simulink model "cav_adas_AutomatedDrivingToolbox"  (R2022a)
settings: Solver=VariableStepAuto  StartTime=0.0  StopTime=500  MaxStep=1e-1  RelTol=1e-3
values from neighbouring files (symbols this model uses):
  Af = 2.33    [data_cav.m]
  Cd = 0.28    [data_cav.m]
  elev_date_1 = date_elev(:,1)    [data_cav.m]
  elev_date_2 = date_elev(:,2)    [data_cav.m]
  eta = 0.93    [data_cav.m]
  fr = 0.015    [data_cav.m]
  g = 9.81    [data_cav.m]
  m = 1521    [data_cav.m]
  R = 0.5    [data_cav.m]
  rho = 1.2    [data_cav.m]
  slope_date_1 = date_slope(:,1)    [data_cav.m]
  slope_date_2_degree = zeros(length(slope_date_2_grad),1)    [data_cav.m]
libraries: sim3dautolib x2, drivingscenarioandsensors x2, mpclib x1, sim3dlib x1
settings Model: Creator=user  LastModifiedBy=user

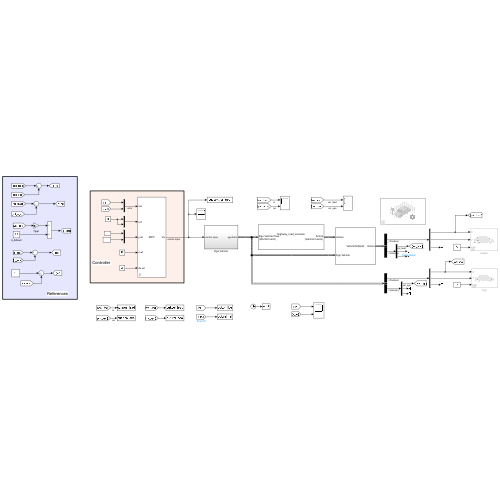
[thumbnail: Simulink's stored preview of the top-level diagram]
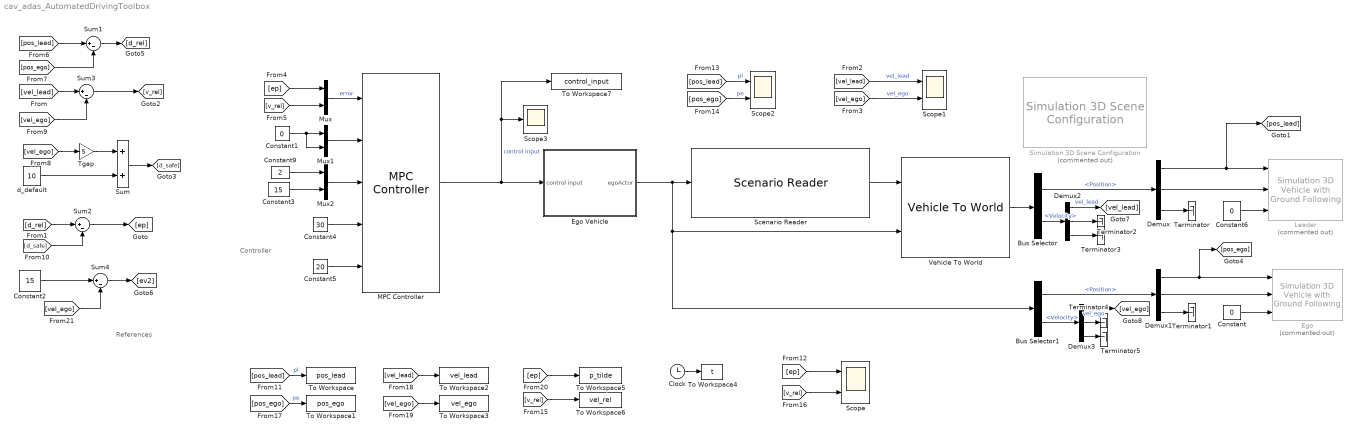
== system cav_adas_AutomatedDrivingToolbox ==
  note: Controller
  note: References
  Bus Selector : BusSelector  OutputSignals=Actors.Position,Actors.Velocity
  Bus Selector1 : BusSelector  OutputSignals=Position,Velocity
  Clock : Clock
  Constant : Constant  Value=0
  Constant1 : Constant  Value=0
  Constant2 : Constant  Value=15
  Constant3 : Constant  Value=15
  Constant4 : Constant  Value=30
  Constant5 : Constant  Value=20
  Constant6 : Constant  Value=0
  Constant9 : Constant  Value=2
  Demux{,1..3} (4 alike) : Demux  Outputs=3
  Ego : sim3dautolib/Simulation 3D Vehicle with Ground Following  Priority=-1  Commented=on  PassVehMesh=Sport utility vehicle  MeshPath=/MathWorksSimulation/Vehicles/Muscle/Meshes/SK_MuscleCar.SK_MuscleCar  TrackWidth=1.9  WheelBase=3  WheelRadius=0.35  VehColor=Blue  InitialPos=[0, 0, 0]  InitialRot=[0, 0, 0]  ActorName=EgoVehicle  SampleTime=-1  ActorType=SimulinkVehicle  ID=C  aMode=3  ActorTag=EgoVehicle  CoordinateScheme=ISO  VehLightsControl=off  HeadlightColor=[ 1, 1, 1 ]  HighBeamIntensity=100000  LowBeamIntensity=60000  HighBeamConeAngle=70  LowBeamConeAngle=70  LeftHeadlightOrientation=[ 0, 0 ]  RightHeadlightOrientation=[ 0, 0 ]  BrakelightIntensity=500  ReverselightIntensity=500  SignallightIntensity=500  SignallightPeriod=1  SignalPulseWidth=50  TransformOutportEnabled=off
      settings: SourceProductBaseCode=VE,AE,DR,UV,VE
  Ego Vehicle : Subsystem
  Leader : sim3dautolib/Simulation 3D Vehicle with Ground Following  Priority=-1  Commented=on  PassVehMesh=Muscle car  MeshPath=/MathWorksSimulation/Vehicles/Muscle/Meshes/SK_MuscleCar.SK_MuscleCar  TrackWidth=1.9  WheelBase=3  WheelRadius=0.35  VehColor=Red  InitialPos=[0, 0, 0]  InitialRot=[0, 0, 0]  ActorName=LeaderVehicle  SampleTime=-1  ActorType=SimulinkVehicle  ID=C  aMode=3  ActorTag=LeaderVehicle  CoordinateScheme=ISO  VehLightsControl=off  HeadlightColor=[ 1, 1, 1 ]  HighBeamIntensity=100000  LowBeamIntensity=60000  HighBeamConeAngle=70  LowBeamConeAngle=70  LeftHeadlightOrientation=[ 0, 0 ]  RightHeadlightOrientation=[ 0, 0 ]  BrakelightIntensity=500  ReverselightIntensity=500  SignallightIntensity=500  SignallightPeriod=1  SignalPulseWidth=50  TransformOutportEnabled=off
      settings: SourceProductBaseCode=VE,AE,DR,UV,VE
  MPC Controller : mpclib/MPC Controller  SCDEnableBlockLinearizationSpecification=on  mpcobj=mpc1  is_multiple=0  enable_value=0  return_u0=off  updateMPCinCallerWorkspace=on  md_inport=off  mv_inport=off  uref_inport=off  return_cost=off  return_mvseq=off  return_qpstatus=off  return_xseq=off  return_state=off  return_ovseq=off  state_inport=off  umin_inport=off  umax_inport=off  ymin_inport=off  ymax_inport=off  cc_inport=off  ywt_inport=on  uwt_inport=on  duwt_inport=on  rhoeps_inport=off  pm_inport=off  MaximumP=10  HorizonChoice=FixedHorizon  n_ts=0.1  n_p=50  n_mv=1  n_md=0  n_ud=0  n_mo=2  n_uo=0  BlockDataType=double  SampleTimeInherited=off  switch_inport=off
  Mux : Mux  Inputs=2
  Mux1 : Mux  Inputs=2
  Mux2 : Mux  Inputs=2
  Scenario Reader : drivingscenarioandsensors/Scenario Reader  ScenarioSource=From file  ScenarioFileName=D:\Università\MAGISTRALE\CSAGV\Challenge 2022\MATLAB & Simulink Files\Highway_road_scenario.mat  ScenarioVariableName=scenario  OutputCoordinateSystem=Vehicle coordinates  EgoVehicleSource=Input port  EgoVehicleActorID=1  OrientVehiclesOnRoad=off  OutputEgoVehiclePose=off  OutputEgoVehicleState=off  SampleTime=0.1  LaneBoundaryOutput=None  LaneBoundaryDistance=0:0.5:9.5  LaneBoundaryLocation=Center of lane markings  BusNameSource=Auto  BusName=BusActors  BusNumActorsSource=Scenario  BusNumActors=100  BusName2Source=Auto  BusName2=BusLaneBoundaries  BusNumLaneBoundariesSource=Scenario  BusNumLaneBoundaries=10  BusName3Source=Auto  BusName3=BusEgoActor  BusName4Source=Auto  BusName4=BusEgoState  ShowCoordinateLabels=on  SimulateUsing=Interpreted execution
  Scope : Scope  NumInputPorts=2
  Scope1 : Scope  NumInputPorts=2
  Scope2 : Scope  NumInputPorts=2
  Scope3 : Scope
  Simulation 3D Scene Configuration : sim3dlib/Simulation 3D Scene Configuration  Priority=0  Commented=on  ProjectFormat=Default Scenes  SceneDesc=Straight road  ProjectName=C:\Program Files\MATLAB\R2022a\toolbox\shared\sim3d_projects\automotive_project\UE4\WindowsNoEditor\VehicleSimulation.exe  ScenePath=/Game/Maps/HwStrght  vehTagList={'EgoVehicle';'LeaderVehicle';'Scene Origin'}  vehTag=EgoVehicle  OpVisEn=off  Ts=1/60  EnableWindow=on  EnableRemoteAccess=off  EnableWeather=off  SunAltitude=40.0  SunAzimuth=90  clouds=10  wind=1  fog=0  rain=0  sensorTag=MainCamera1  sensorId=1  sensorName=MainCamera1  mountLoc=Origin  offsetFlag=off  tmountOffset=[0, 0, 0]  rmountOffset=[0, 0, 0]  HorizontalResolution=1280  VerticalResolution=720  HorizontalFOV=60  mountPoint=[0 0 0]  mountOrientation=[0 0 0]  aMode=3  ID=1
      settings: SourceProductBaseCode=VE,AE,DR,UV,VE
  Sum : Sum
  Sum{1..4} (4 alike) : Sum  Inputs=|+-
  Terminator{,1..5} (6 alike) : Terminator
  Tgap : Gain  Gain=5
  To Workspace : ToWorkspace  VariableName=pos_lead  SampleTime=-1
      settings: Save2DSignal=2-D array (concatenate along first dimension)
  To Workspace1 : ToWorkspace  VariableName=pos_ego  SampleTime=-1
      settings: Save2DSignal=2-D array (concatenate along first dimension)
  To Workspace2 : ToWorkspace  VariableName=vel_lead  SampleTime=-1
      settings: Save2DSignal=2-D array (concatenate along first dimension)
  To Workspace3 : ToWorkspace  VariableName=vel_ego  SampleTime=-1
      settings: Save2DSignal=2-D array (concatenate along first dimension)
  To Workspace4 : ToWorkspace  VariableName=t  SampleTime=-1
      settings: Save2DSignal=2-D array (concatenate along first dimension)
  To Workspace5 : ToWorkspace  VariableName=p_tilde  SampleTime=-1
      settings: Save2DSignal=2-D array (concatenate along first dimension)
  To Workspace6 : ToWorkspace  VariableName=vel_rel  SampleTime=-1
      settings: Save2DSignal=2-D array (concatenate along first dimension)
  To Workspace7 : ToWorkspace  VariableName=control_input  SampleTime=-1
      settings: Save2DSignal=2-D array (concatenate along first dimension)
  Vehicle To World : drivingscenarioandsensors/Vehicle To World  BusNameSource=Auto  BusName=BusVehicleToWorldActors  SimulateUsing=Interpreted execution
      settings: SourceProductBaseCode=DR
  d_default : Constant  Value=10
  wires:
  Mux1/1 -> MPC Controller/2
  [d_safe] -> Sum2/2
  [d_rel] -> Sum2/1
  Sum2/1 -> [ep]
  Sum/1 -> [d_safe]
  Mux2/1 -> MPC Controller/3
  [ep] -> Mux/1
  d_default/1 -> Sum/2
  Constant1/1 -> Mux1/2, Mux1/1
  Constant3/1 -> Mux2/2
  Constant5/1 -> MPC Controller/5
  [vel_ego] -> Sum3/2
  Tgap/1 -> Sum/1
  Sum3/1 -> [v_rel]
  Mux/1 -> MPC Controller/1  "error"
  [vel_ego] -> Tgap/1
  [pos_lead] -> Scope2/1  "pl"
  Constant4/1 -> MPC Controller/4
  [pos_ego] -> Sum1/2
  [vel_ego] -> Scope1/2  "vel_ego"
  [vel_lead] -> Scope1/1  "vel_lead"
  Sum1/1 -> [d_rel]
  [pos_ego] -> Scope2/2  "pe"
  Ego Vehicle/1(egoActor) -> Bus Selector1/1, Vehicle To World/2, Scenario Reader/1
  Scenario Reader/1 -> Vehicle To World/1
  Vehicle To World/1 -> Bus Selector/1
  Bus Selector/1 -> Demux/1  "<Position>"
  Bus Selector1/1 -> Demux1/1  "<Position>"
  Constant/1 -> Ego/3
  Constant6/1 -> Leader/3
  Demux/3 -> Terminator/1
  Demux/1 -> Leader/1, [pos_lead]
  Demux/2 -> Leader/2
  Demux1/3 -> Terminator1/1
  Demux1/1 -> Ego/1, [pos_ego]
  Demux1/2 -> Ego/2
  Bus Selector/2 -> Demux2/1  "<Velocity>"
  Bus Selector1/2 -> Demux3/1  "<Velocity>"
  Demux2/1 -> [vel_lead]  "vel_lead"
  Demux2/2 -> Terminator2/1
  Demux2/3 -> Terminator3/1
  Demux3/2 -> Terminator4/1
  Demux3/3 -> Terminator5/1
  Demux3/1 -> [vel_ego]  "vel_ego"
  MPC Controller/1 -> Scope3/1, To Workspace7/1, Ego Vehicle/1(control input)  "control input"
  [vel_lead] -> Sum3/1
  [pos_lead] -> Sum1/1
  [v_rel] -> Mux/2
  Constant9/1 -> Mux2/1
  [v_rel] -> To Workspace6/1
  [pos_ego] -> To Workspace1/1  "pe"
  [pos_lead] -> To Workspace/1  "pl"
  [vel_ego] -> To Workspace3/1
  [ep] -> To Workspace5/1
  [vel_lead] -> To Workspace2/1
  Clock/1 -> To Workspace4/1
  [v_rel] -> Scope/2
  [ep] -> Scope/1
  Sum4/1 -> [ev2]
  Constant2/1 -> Sum4/1
  [vel_ego] -> Sum4/2

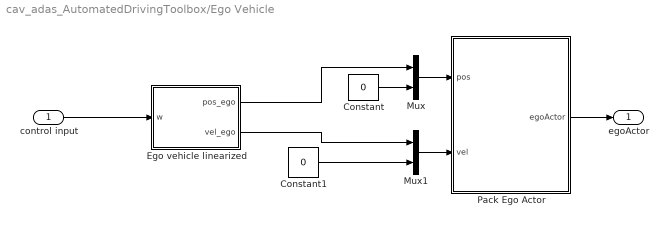
== system cav_adas_AutomatedDrivingToolbox/Ego Vehicle ==
  control input : Inport
  Constant : Constant  Value=0
  Constant1 : Constant  Value=0
  Ego vehicle linearized : Subsystem
  Mux : Mux  Inputs=2
  Mux1 : Mux  Inputs=2
  Pack Ego Actor : MATLAB Function  TreatAsAtomicUnit=on
  egoActor : Outport
  wires:
  control input/1 -> Ego vehicle linearized/1(w)
  Pack Ego Actor/1(egoActor) -> egoActor/1
  Mux/1 -> Pack Ego Actor/1(pos)
  Mux1/1 -> Pack Ego Actor/2(vel)
  Ego vehicle linearized/1(pos_ego) -> Mux/1
  Ego vehicle linearized/2(vel_ego) -> Mux1/1
  Constant1/1 -> Mux1/2
  Constant/1 -> Mux/2

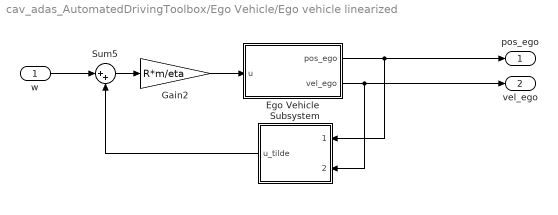
== system cav_adas_AutomatedDrivingToolbox/Ego Vehicle/Ego vehicle linearized ==
  w : Inport
  "Ego Vehicle " : Subsystem
  Gain2 : Gain  Gain=R*m/eta
  Subsystem : Subsystem
  Sum5 : Sum  Inputs=|++
  pos_ego : Outport
  vel_ego : Outport  Port=2
  wires:
  "Ego Vehicle "/2(vel_ego) -> vel_ego/1, Subsystem/2(vel_ego)
  "Ego Vehicle "/1(pos_ego) -> pos_ego/1, Subsystem/1(pos_ego)
  Sum5/1 -> Gain2/1
  w/1 -> Sum5/1
  Gain2/1 -> "Ego Vehicle "/1(u)
  Subsystem/1(u_tilde) -> Sum5/2

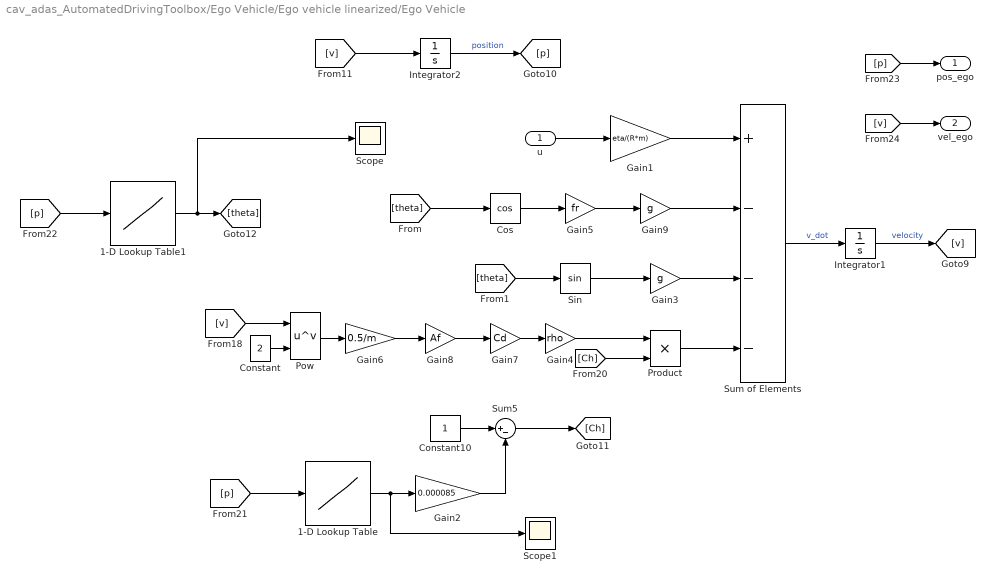
== system cav_adas_AutomatedDrivingToolbox/Ego Vehicle/Ego vehicle linearized/Ego Vehicle  ==
  u : Inport
  1-D Lookup Table : Lookup_n-D  NumberOfTableDimensions=1  BreakpointsForDimension1=elev_date_1  Table=elev_date_2  InternalRulePriority=Speed  RndMeth=Simplest
  1-D Lookup Table1 : Lookup_n-D  NumberOfTableDimensions=1  BreakpointsForDimension1=slope_date_1  Table=slope_date_2_degree  InternalRulePriority=Speed  RndMeth=Simplest
  Constant : Constant  Value=2
  Constant10 : Constant
  Cos : Trigonometry  Operator=cos
  Gain1 : Gain  Gain=eta/(R*m)
  Gain2 : Gain  Gain=0.000085
  Gain3 : Gain  Gain=g
  Gain4 : Gain  Gain=rho
  Gain5 : Gain  Gain=fr
  Gain6 : Gain  Gain=0.5/m
  Gain7 : Gain  Gain=Cd
  Gain8 : Gain  Gain=Af
  Gain9 : Gain  Gain=g
  Integrator1 : Integrator
  Integrator2 : Integrator
  Pow : Math  Operator=pow  RndMeth=Zero
  Product : Product
  Scope : Scope
  Scope1 : Scope
  Sin : Trigonometry
  Sum of Elements : Sum  Inputs=+---
  Sum5 : Sum  Inputs=|+-
  pos_ego : Outport
  vel_ego : Outport  Port=2
  wires:
  [p] -> 1-D Lookup Table/1
  1-D Lookup Table1/1 -> Scope/1, [theta]
  Gain5/1 -> Gain9/1
  Gain6/1 -> Gain8/1
  [Ch] -> Product/2
  Sin/1 -> Gain3/1
  Gain4/1 -> Product/1
  Sum5/1 -> [Ch]
  Gain1/1 -> Sum of Elements/1
  Integrator2/1 -> [p]  "position"
  Constant10/1 -> Sum5/1
  Gain9/1 -> Sum of Elements/2
  Integrator1/1 -> [v]  "velocity"
  Pow/1 -> Gain6/1
  Gain8/1 -> Gain7/1
  Gain2/1 -> Sum5/2
  Cos/1 -> Gain5/1
  Sum of Elements/1 -> Integrator1/1  "v_dot"
  1-D Lookup Table/1 -> Scope1/1, Gain2/1
  Gain7/1 -> Gain4/1
  [v] -> vel_ego/1
  [v] -> Integrator2/1
  Constant/1 -> Pow/2
  [p] -> 1-D Lookup Table1/1
  [v] -> Pow/1
  Gain3/1 -> Sum of Elements/3
  [p] -> pos_ego/1
  Product/1 -> Sum of Elements/4
  u/1 -> Gain1/1
  [theta] -> Cos/1
  [theta] -> Sin/1

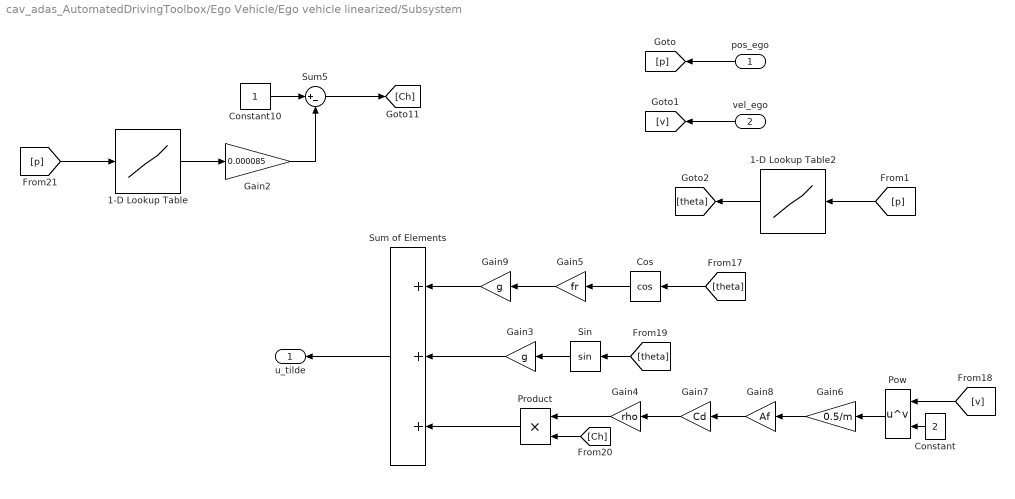
== system cav_adas_AutomatedDrivingToolbox/Ego Vehicle/Ego vehicle linearized/Subsystem ==
  pos_ego : Inport
  vel_ego : Inport  Port=2
  1-D Lookup Table : Lookup_n-D  NumberOfTableDimensions=1  BreakpointsForDimension1=elev_date_1  Table=elev_date_2  InternalRulePriority=Speed  RndMeth=Simplest
  1-D Lookup Table2 : Lookup_n-D  NumberOfTableDimensions=1  BreakpointsForDimension1=slope_date_1  Table=slope_date_2_degree  InternalRulePriority=Speed  RndMeth=Simplest
  Constant : Constant  Value=2
  Constant10 : Constant
  Cos : Trigonometry  Operator=cos
  Gain2 : Gain  Gain=0.000085
  Gain3 : Gain  Gain=g
  Gain4 : Gain  Gain=rho
  Gain5 : Gain  Gain=fr
  Gain6 : Gain  Gain=0.5/m
  Gain7 : Gain  Gain=Cd
  Gain8 : Gain  Gain=Af
  Gain9 : Gain  Gain=g
  Pow : Math  Operator=pow  RndMeth=Zero
  Product : Product
  Sin : Trigonometry
  Sum of Elements : Sum  Inputs=+++
  Sum5 : Sum  Inputs=|+-
  u_tilde : Outport
  wires:
  pos_ego/1 -> [p]
  vel_ego/1 -> [v]
  Cos/1 -> Gain5/1
  Sin/1 -> Gain3/1
  Gain7/1 -> Gain4/1
  [v] -> Pow/1
  Gain8/1 -> Gain7/1
  Gain6/1 -> Gain8/1
  Constant/1 -> Pow/2
  Pow/1 -> Gain6/1
  Gain4/1 -> Product/1
  [Ch] -> Product/2
  [theta] -> Sin/1
  Gain5/1 -> Gain9/1
  [p] -> 1-D Lookup Table2/1
  1-D Lookup Table2/1 -> [theta]
  1-D Lookup Table/1 -> Gain2/1
  Gain2/1 -> Sum5/2
  [p] -> 1-D Lookup Table/1
  Constant10/1 -> Sum5/1
  Sum5/1 -> [Ch]
  Sum of Elements/1 -> u_tilde/1
  [theta] -> Cos/1
  Gain9/1 -> Sum of Elements/1
  Gain3/1 -> Sum of Elements/2
  Product/1 -> Sum of Elements/3

== matlab function cav_adas_AutomatedDrivingToolbox/Ego Vehicle/Pack Ego Actor ==
  data: pos input; egoActor output Bus: BusActors1Actors size=1; vel input
function egoActor = packEgo(pos,vel)

egoActor = struct(...
    'ActorID',1,...
    'Position', [pos(1) pos(2) 0], ...
    'Velocity', [vel(1) vel(2) 0], ...
    'Roll', 0, ...
    'Pitch', 0, ...
    'Yaw', 0, ...
    'AngularVelocity', [0 0 0]);
end
